simulink model "Calibrate_InputDevice"  (R2025b)
settings: Solver=VariableStepAuto  StartTime=0.0  StopTime=inf  RelTol=1e-3
libraries: sl3dlib x1
settings Model: Creator=klakhara  LastModifiedBy=klakhara

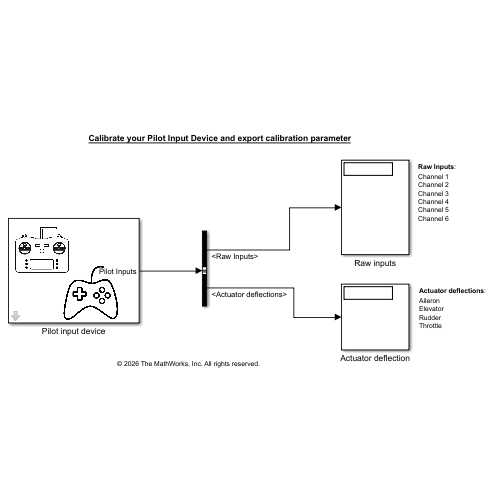
[thumbnail: Simulink's stored preview of the top-level diagram]
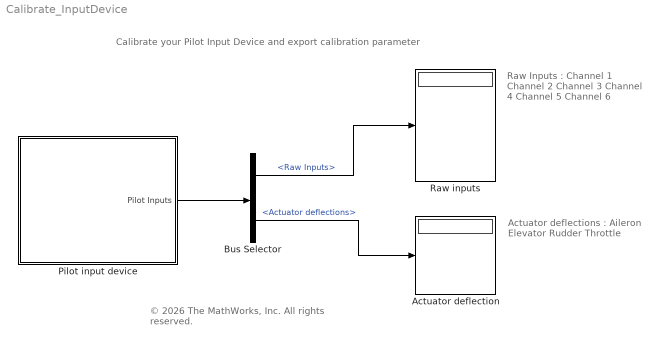
== system Calibrate_InputDevice ==
  note: © 2026 The MathWorks, Inc. All rights reserved.
  note: Calibrate your Pilot Input Device and export calibration parameter
  note: Actuator deflections :
      | Aileron
      | Elevator
      | Rudder
      | Throttle
  note: Raw Inputs :
      | Channel 1
      | Channel 2
      | Channel 3
      | Channel 4
      | Channel 5
      | Channel 6
  Actuator deflection : Display
  Bus Selector : BusSelector  OutputSignals=Raw Inputs,Actuator deflections
  Pilot input device : Subsystem  mask{joystickID=Joystick1, rollCh=6, uRollMin=0.0873, uRollMax=0.9173, rollDB=0.5, dirRoll=on, pitchCh=2, uPitchMin=-0.8347, uPitchMax=0.8254, pitchDB=0.07, dirPitch=off, yawCh=1, uYawMin=-0.8347, uYawMax=0.8254, yawDB=0.1, dirYaw=off, throttleCh=3, uThrottleMin=0.02777, uThrottleMax=0.9961, throttleDB=0.05, dirThrottle=off, aileronMin=-15, aileronMax=15, elevatorMin=-25, elevatorMax=25, rudderMin=-20, rudderMax=20}
      mask prompts: joystickID "Device ID:"; rollCh "Channel:"; uRollMin "uMin:"; uRollMax "uMax:"; rollDB "Deadband:"; dirRoll "Reverse direction"; pitchCh "Channel:"; uPitchMin "uMin:"; uPitchMax "uMax:"; pitchDB "Deadband:"; dirPitch "Reverse direction"; yawCh "Channel:"; uYawMin "uMin:"; uYawMax "uMax:"; yawDB "Deadband:"; dirYaw "Reverse direction"; throttleCh "Channel:"; uThrottleMin "uMin:"; uThrottleMax "uMax:"; throttleDB "Deadband:"; dirThrottle "Reverse direction"; aileronMin "Min(°):"; aileronMax "Max(°):"; elevatorMin "Min(°):"; elevatorMax "Max(°):"; rudderMin "Min(°):"; rudderMax "Max(°):"
      mask TypeOptions joystickID: None | Joystick1 | Joystick2 | Joystick3 | Joystick4 | Joystick5 | Joystick6 | Joystick7 | Joystick8 | Joystick9 | Joystick10 | Joystick11 | Joystick12
      mask TypeOptions rollCh: 1 | 2 | 3 | 4 | 5 | 6
      mask TypeOptions pitchCh: 1 | 2 | 3 | 4 | 5 | 6
      mask TypeOptions yawCh: 1 | 2 | 3 | 4 | 5 | 6
      mask TypeOptions throttleCh: 1 | 2 | 3 | 4 | 5 | 6
      mask DialogControl DescGroupVar Prompt: Set up and calibrate your Pilot Input Device
      mask DialogControl DescTextVar Prompt: Use this subsystem to set up and calibrate your pilot input device.  You can also export the calibration parameters once you get the adequate outputs in the ‘Actuator deflection’ display.
      mask DialogControl ParameterGroupVar Prompt: Identify your pilot input device:
      mask DialogControl Control10 Prompt: Connect your pilot input device (Joystick/ RC Controller/ Flying Stick),  via USB and select your device ID.
      mask DialogControl Container4 Prompt: Set up your control limits:
      mask DialogControl Control15 Prompt: For each control surface, mention its maximum and minimum deflections.
      mask DialogControl Control6 Prompt: Aileron:
      mask DialogControl Control6_copy Prompt: Elevator:
      mask DialogControl Control6_copy_copy Prompt: Rudder:
      mask DialogControl Container3 Prompt: Calibrate your channels:
      mask DialogControl Control10_copy Prompt: Connect your pilot input device (Joystick/ RC Controller/ Flying Stick),  via USB and select your controller ID.
      mask DialogControl Control13 Prompt: uMin and uMax: Once the channel is selected, move the sticks to the extreme and identify the max and min values, and accordingly populate uMin and uMax.
      mask DialogControl Control12 Prompt: Channel: Deflect the control sticks/press the buttons one by one on the Pilot Input Device, and identify the channel number at which the values change. For each control, identify the channel number and select from the dropdown.
      mask DialogControl Control14 Prompt: Deadband:  In case your controller is providing a residual value,  at the mid position where zero is desired. It is advised to use residual value + 0.01 as the deadband value.
      mask DialogControl Control16 Prompt: Reverse direction: Check the box to change the actuator deflection directions.
      mask DialogControl Control2 Prompt: Roll:
      mask DialogControl Control3 Prompt: Pitch:
      mask DialogControl Control4 Prompt: Yaw:
      mask DialogControl Control5 Prompt: Throttle
      mask DialogControl Container5 Prompt: Export Calibration parameters:
      mask DialogControl saveConfig Prompt: Export
      mask Display: image('Controller_Setup.jpg');
  Raw inputs : Display
  wires:
  Pilot input device/1(Pilot Inputs) -> Bus Selector/1
  Bus Selector/1 -> Raw inputs/1  "<Raw Inputs>"
  Bus Selector/2 -> Actuator deflection/1  "<Actuator deflections>"

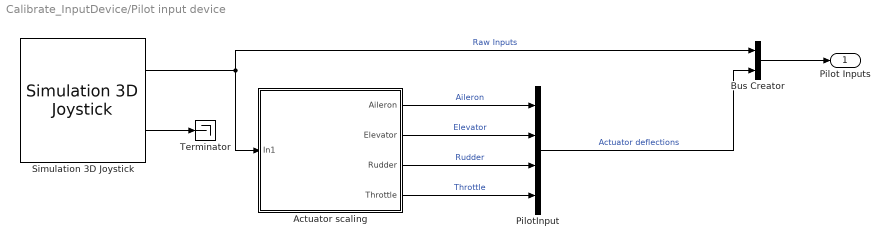
== system Calibrate_InputDevice/Pilot input device ==
  Actuator scaling : Subsystem
  Bus Creator : BusCreator  Inputs=2
  PilotInput : BusCreator  Inputs=4
  Simulation 3D Joystick : sl3dlib/Simulation 3D/Hardware Interface/Simulation 3D Joystick  joyid=1  adjustports=on  forcefeed=off
  Terminator : Terminator
  Pilot Inputs : Outport
  wires:
  Bus Creator/1 -> Pilot Inputs/1
  Simulation 3D Joystick/1 -> Actuator scaling/1(In1), Bus Creator/1  "Raw Inputs"
  Actuator scaling/2(Elevator) -> PilotInput/2  "Elevator"
  Simulation 3D Joystick/2 -> Terminator/1
  PilotInput/1 -> Bus Creator/2  "Actuator deflections"
  Actuator scaling/3(Rudder) -> PilotInput/3  "Rudder"
  Actuator scaling/4(Throttle) -> PilotInput/4  "Throttle"
  Actuator scaling/1(Aileron) -> PilotInput/1  "Aileron"

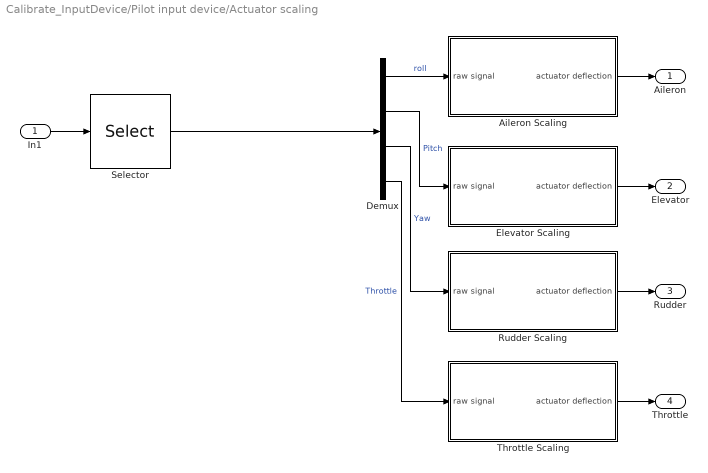
== system Calibrate_InputDevice/Pilot input device/Actuator scaling ==
  In1 : Inport
  Aileron Scaling : Subsystem
  Demux : Demux
  Elevator Scaling : Subsystem
  Rudder Scaling : Subsystem
  Selector : Selector  IndexOptions=Index vector (dialog)  Indices=[rollCh pitchCh yawCh throttleCh]  OutputSizes=1
  Throttle Scaling : Subsystem
  Aileron : Outport
  Elevator : Outport  Port=2
  Rudder : Outport  Port=3
  Throttle : Outport  Port=4
  wires:
  In1/1 -> Selector/1
  Rudder Scaling/1(actuator deflection) -> Rudder/1
  Demux/3 -> Rudder Scaling/1(raw signal)  "Yaw"
  Demux/1 -> Aileron Scaling/1(raw signal)  "roll"
  Selector/1 -> Demux/1
  Elevator Scaling/1(actuator deflection) -> Elevator/1
  Demux/4 -> Throttle Scaling/1(raw signal)  "Throttle"
  Demux/2 -> Elevator Scaling/1(raw signal)  "Pitch"
  Aileron Scaling/1(actuator deflection) -> Aileron/1
  Throttle Scaling/1(actuator deflection) -> Throttle/1

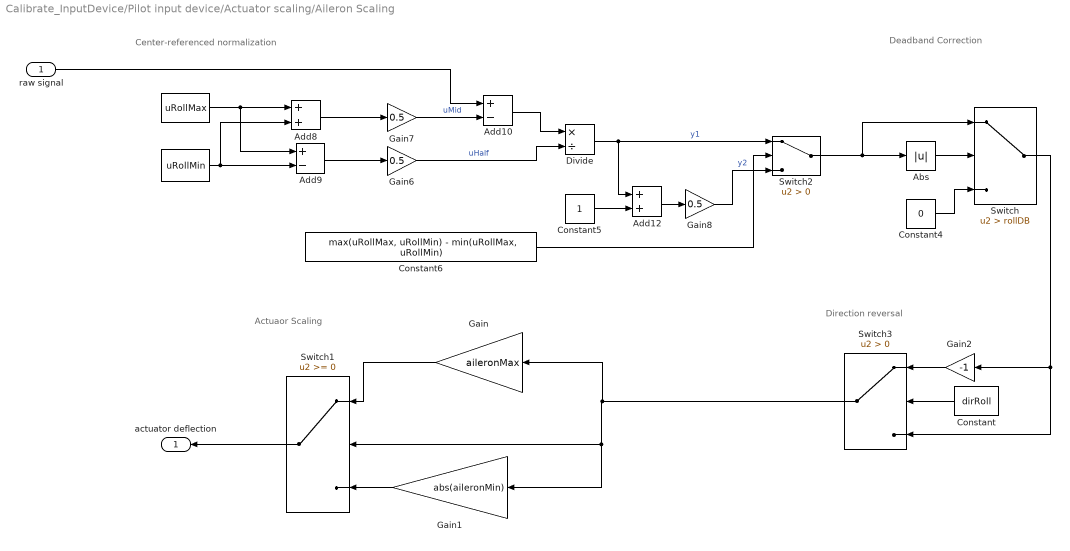
== system Calibrate_InputDevice/Pilot input device/Actuator scaling/Aileron Scaling ==
  note: Direction reversal
  note: Center-referenced normalization
  note: Deadband Correction
  note: Actuaor Scaling
  raw signal : Inport
  " " : Constant  Value=uRollMin
  "   " : Constant  Value=uRollMax
  Abs : Abs  SaturateOnIntegerOverflow=off
  Add10 : Sum  Inputs=+-
  Add12 : Sum
  Add8 : Sum
  Add9 : Sum  Inputs=+-
  Constant : Constant  Value=dirRoll
  Constant4 : Constant  Value=0
  Constant5 : Constant
  Constant6 : Constant  Value=max(uRollMax, uRollMin) - min(uRollMax, uRollMin)
  Divide : Product  Inputs=*/
  Gain : Gain  Gain=aileronMax
  Gain1 : Gain  Gain=abs(aileronMin)
  Gain2 : Gain  Gain=-1
  Gain6 : Gain  Gain=0.5
  Gain7 : Gain  Gain=0.5
  Gain8 : Gain  Gain=0.5
  Switch : Switch  Criteria=u2 > Threshold  Threshold=rollDB  SaturateOnIntegerOverflow=off  InputSameDT=off
  Switch1 : Switch  SaturateOnIntegerOverflow=off  InputSameDT=off
  Switch2 : Switch  Criteria=u2 > Threshold  SaturateOnIntegerOverflow=off  InputSameDT=off
  Switch3 : Switch  Criteria=u2 > Threshold  SaturateOnIntegerOverflow=off  InputSameDT=off
  actuator deflection : Outport
  wires:
  Add9/1 -> Gain6/1
  "   "/1 -> Add9/1, Add8/1
  Add8/1 -> Gain7/1
  " "/1 -> Add8/2, Add9/2
  raw signal/1 -> Add10/1
  Gain7/1 -> Add10/2  "uMid"
  Add10/1 -> Divide/1
  Gain6/1 -> Divide/2  "uHalf"
  Switch1/1 -> actuator deflection/1
  Divide/1 -> Add12/1, Switch2/1  "y1"
  Constant5/1 -> Add12/2
  Add12/1 -> Gain8/1
  Constant6/1 -> Switch2/2
  Gain8/1 -> Switch2/3  "y2"
  Abs/1 -> Switch/2
  Constant4/1 -> Switch/3
  Switch/1 -> Gain2/1, Switch3/3
  Gain/1 -> Switch1/1
  Gain1/1 -> Switch1/3
  Gain2/1 -> Switch3/1
  Switch3/1 -> Gain1/1, Switch1/2, Gain/1
  Constant/1 -> Switch3/2
  Switch2/1 -> Switch/1, Abs/1

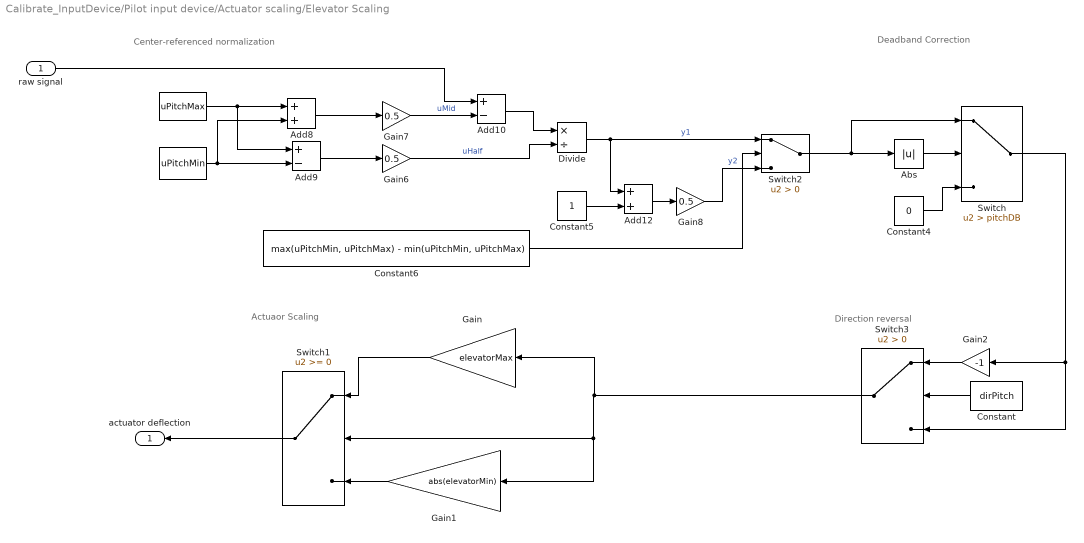
== system Calibrate_InputDevice/Pilot input device/Actuator scaling/Elevator Scaling ==
  note: Direction reversal
  note: Center-referenced normalization
  note: Deadband Correction
  note: Actuaor Scaling
  raw signal : Inport
  " " : Constant  Value=uPitchMin
  "   " : Constant  Value=uPitchMax
  Abs : Abs  SaturateOnIntegerOverflow=off
  Add10 : Sum  Inputs=+-
  Add12 : Sum
  Add8 : Sum
  Add9 : Sum  Inputs=+-
  Constant : Constant  Value=dirPitch
  Constant4 : Constant  Value=0
  Constant5 : Constant
  Constant6 : Constant  Value=max(uPitchMin, uPitchMax) - min(uPitchMin, uPitchMax)
  Divide : Product  Inputs=*/
  Gain : Gain  Gain=elevatorMax
  Gain1 : Gain  Gain=abs(elevatorMin)
  Gain2 : Gain  Gain=-1
  Gain6 : Gain  Gain=0.5
  Gain7 : Gain  Gain=0.5
  Gain8 : Gain  Gain=0.5
  Switch : Switch  Criteria=u2 > Threshold  Threshold=pitchDB  SaturateOnIntegerOverflow=off  InputSameDT=off
  Switch1 : Switch  SaturateOnIntegerOverflow=off  InputSameDT=off
  Switch2 : Switch  Criteria=u2 > Threshold  SaturateOnIntegerOverflow=off  InputSameDT=off
  Switch3 : Switch  Criteria=u2 > Threshold  SaturateOnIntegerOverflow=off  InputSameDT=off
  actuator deflection : Outport
  wires:
  Add9/1 -> Gain6/1
  "   "/1 -> Add9/1, Add8/1
  Add8/1 -> Gain7/1
  " "/1 -> Add8/2, Add9/2
  raw signal/1 -> Add10/1
  Gain7/1 -> Add10/2  "uMid"
  Add10/1 -> Divide/1
  Gain6/1 -> Divide/2  "uHalf"
  Switch1/1 -> actuator deflection/1
  Divide/1 -> Add12/1, Switch2/1  "y1"
  Constant5/1 -> Add12/2
  Add12/1 -> Gain8/1
  Constant6/1 -> Switch2/2
  Gain8/1 -> Switch2/3  "y2"
  Abs/1 -> Switch/2
  Constant4/1 -> Switch/3
  Switch/1 -> Gain2/1, Switch3/3
  Gain/1 -> Switch1/1
  Gain1/1 -> Switch1/3
  Gain2/1 -> Switch3/1
  Switch3/1 -> Gain1/1, Switch1/2, Gain/1
  Constant/1 -> Switch3/2
  Switch2/1 -> Switch/1, Abs/1

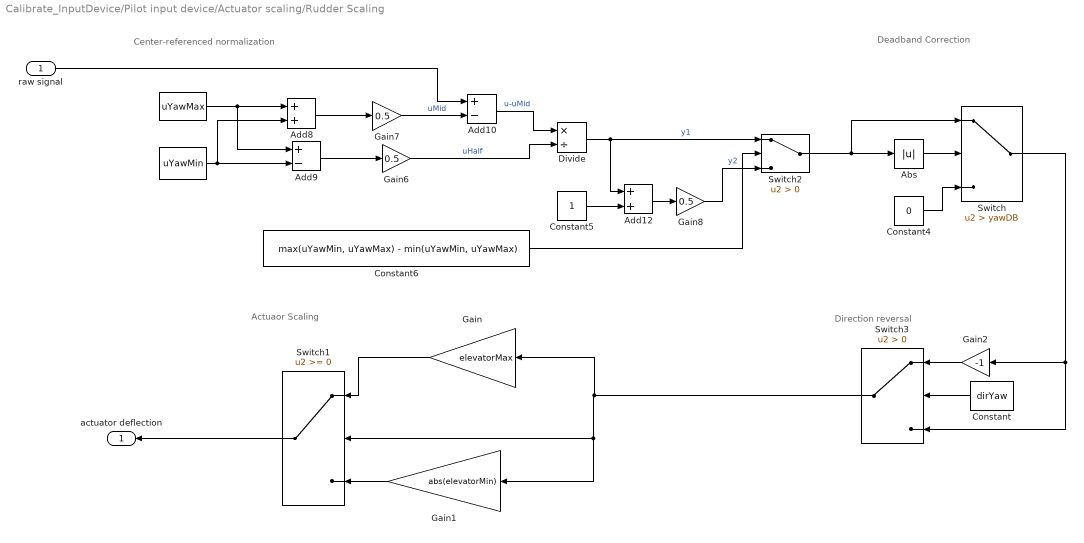
== system Calibrate_InputDevice/Pilot input device/Actuator scaling/Rudder Scaling ==
  note: Direction reversal
  note: Center-referenced normalization
  note: Deadband Correction
  note: Actuaor Scaling
  raw signal : Inport
  " " : Constant  Value=uYawMin
  "   " : Constant  Value=uYawMax
  Abs : Abs  SaturateOnIntegerOverflow=off
  Add10 : Sum  Inputs=+-
  Add12 : Sum
  Add8 : Sum
  Add9 : Sum  Inputs=+-
  Constant : Constant  Value=dirYaw
  Constant4 : Constant  Value=0
  Constant5 : Constant
  Constant6 : Constant  Value=max(uYawMin, uYawMax) - min(uYawMin, uYawMax)
  Divide : Product  Inputs=*/
  Gain : Gain  Gain=elevatorMax
  Gain1 : Gain  Gain=abs(elevatorMin)
  Gain2 : Gain  Gain=-1
  Gain6 : Gain  Gain=0.5
  Gain7 : Gain  Gain=0.5
  Gain8 : Gain  Gain=0.5
  Switch : Switch  Criteria=u2 > Threshold  Threshold=yawDB  SaturateOnIntegerOverflow=off  InputSameDT=off
  Switch1 : Switch  SaturateOnIntegerOverflow=off  InputSameDT=off
  Switch2 : Switch  Criteria=u2 > Threshold  SaturateOnIntegerOverflow=off  InputSameDT=off
  Switch3 : Switch  Criteria=u2 > Threshold  SaturateOnIntegerOverflow=off  InputSameDT=off
  actuator deflection : Outport
  wires:
  Add9/1 -> Gain6/1
  "   "/1 -> Add9/1, Add8/1
  Add8/1 -> Gain7/1
  " "/1 -> Add8/2, Add9/2
  raw signal/1 -> Add10/1
  Gain7/1 -> Add10/2  "uMid"
  Add10/1 -> Divide/1  "u-uMid"
  Gain6/1 -> Divide/2  "uHalf"
  Switch1/1 -> actuator deflection/1
  Divide/1 -> Add12/1, Switch2/1  "y1"
  Constant5/1 -> Add12/2
  Add12/1 -> Gain8/1
  Constant6/1 -> Switch2/2
  Gain8/1 -> Switch2/3  "y2"
  Abs/1 -> Switch/2
  Constant4/1 -> Switch/3
  Switch/1 -> Gain2/1, Switch3/3
  Gain/1 -> Switch1/1
  Gain1/1 -> Switch1/3
  Gain2/1 -> Switch3/1
  Switch3/1 -> Gain1/1, Switch1/2, Gain/1
  Constant/1 -> Switch3/2
  Switch2/1 -> Switch/1, Abs/1

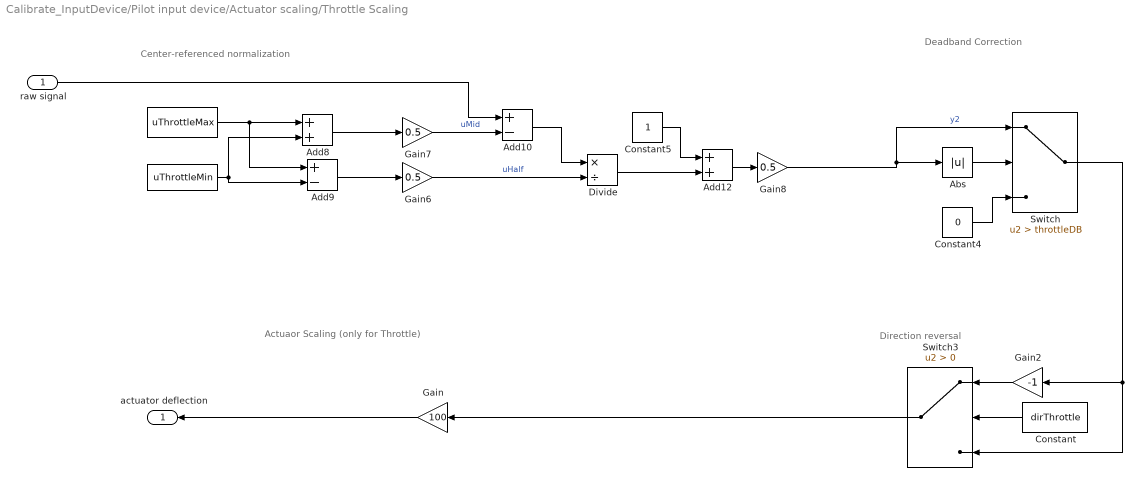
== system Calibrate_InputDevice/Pilot input device/Actuator scaling/Throttle Scaling ==
  note: Direction reversal
  note: Center-referenced normalization
  note: Deadband Correction
  note: Actuaor Scaling (only for Throttle)
  raw signal : Inport
  " " : Constant  Value=uThrottleMin
  "   " : Constant  Value=uThrottleMax
  Abs : Abs  SaturateOnIntegerOverflow=off
  Add10 : Sum  Inputs=+-
  Add12 : Sum
  Add8 : Sum
  Add9 : Sum  Inputs=+-
  Constant : Constant  Value=dirThrottle
  Constant4 : Constant  Value=0
  Constant5 : Constant
  Divide : Product  Inputs=*/
  Gain : Gain  Gain=100
  Gain2 : Gain  Gain=-1
  Gain6 : Gain  Gain=0.5
  Gain7 : Gain  Gain=0.5
  Gain8 : Gain  Gain=0.5
  Switch : Switch  Criteria=u2 > Threshold  Threshold=throttleDB  SaturateOnIntegerOverflow=off  InputSameDT=off
  Switch3 : Switch  Criteria=u2 > Threshold  SaturateOnIntegerOverflow=off  InputSameDT=off
  actuator deflection : Outport
  wires:
  Add9/1 -> Gain6/1
  "   "/1 -> Add9/1, Add8/1
  Add8/1 -> Gain7/1
  " "/1 -> Add9/2, Add8/2
  raw signal/1 -> Add10/1
  Gain7/1 -> Add10/2  "uMid"
  Add10/1 -> Divide/1
  Gain6/1 -> Divide/2  "uHalf"
  Add12/1 -> Gain8/1
  Gain8/1 -> Switch/1, Abs/1  "y2"
  Abs/1 -> Switch/2
  Constant4/1 -> Switch/3
  Switch/1 -> Gain2/1, Switch3/3
  Gain2/1 -> Switch3/1
  Constant/1 -> Switch3/2
  Gain/1 -> actuator deflection/1
  Switch3/1 -> Gain/1
  Constant5/1 -> Add12/1
  Divide/1 -> Add12/2
